simulink model "model"  (R2014a)
settings: Solver=ode45  StartTime=0.0  StopTime=30  RelTol=1e-3
undefined symbols (not defined in the file or in its folder): G0_den, G0_num, Gc_den, Gc_num
libraries: simulink x2
settings Model: Creator=Jian  LastModifiedBy=Jian

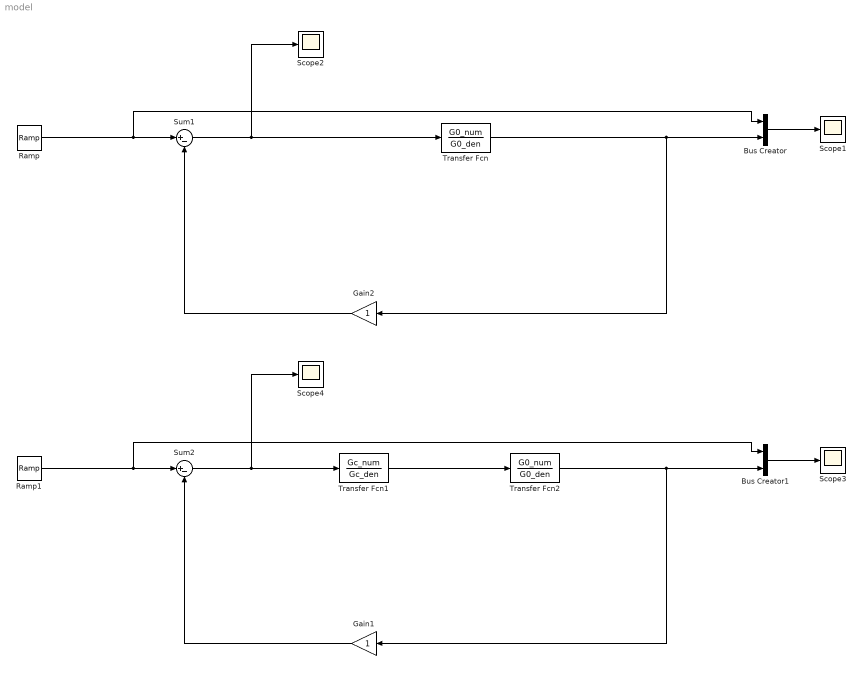
== system model ==
  Bus Creator : BusCreator  Inputs=2
  Bus Creator1 : BusCreator  Inputs=2
  Gain1 : Gain
  Gain2 : Gain
  Ramp : simulink/Sources/Ramp  slope=1  start=0  X0=0
  Ramp1 : simulink/Sources/Ramp  slope=1  start=0  X0=0
  Scope{1..4} (4 alike) : Scope
      Scope1 settings: TimeRange=10  MaxDataPoints=500000
      Scope2 settings: TimeRange=10  MaxDataPoints=500000
      Scope3 settings: TimeRange=10  SaveName=ScopeData2  MaxDataPoints=500000
      Scope4 settings: TimeRange=10  SaveName=ScopeData3  MaxDataPoints=500000
  Sum1 : Sum  Inputs=|+-
  Sum2 : Sum  Inputs=|+-
  Transfer Fcn : TransferFcn  Numerator=G0_num  Denominator=G0_den
  Transfer Fcn1 : TransferFcn  Numerator=Gc_num  Denominator=Gc_den
  Transfer Fcn2 : TransferFcn  Numerator=G0_num  Denominator=G0_den
  wires:
  Ramp/1 -> Bus Creator/1, Sum1/1
  Transfer Fcn/1 -> Gain2/1, Bus Creator/2
  Gain2/1 -> Sum1/2
  Bus Creator/1 -> Scope1/1
  Sum1/1 -> Scope2/1, Transfer Fcn/1
  Ramp1/1 -> Bus Creator1/1, Sum2/1
  Transfer Fcn1/1 -> Transfer Fcn2/1
  Gain1/1 -> Sum2/2
  Bus Creator1/1 -> Scope3/1
  Sum2/1 -> Scope4/1, Transfer Fcn1/1
  Transfer Fcn2/1 -> Gain1/1, Bus Creator1/2
